simulink model "physicalModel"  (R2020b)
settings: Solver=ode3  StartTime=0.0  StopTime=10.0  FixedStep=Ts  RelTol=1e-3  EnableMultiTasking=on
undefined symbols (not defined in the file): Earth, init, Vehicle, WGS84
libraries: dynamicsLibrary x4, shared6dof x1, aerolibtransform2 x1
settings Model: Creator=dbell44  LastModifiedBy=dbell44
settings DebuggingCC: BusObjectLabelMismatch=none

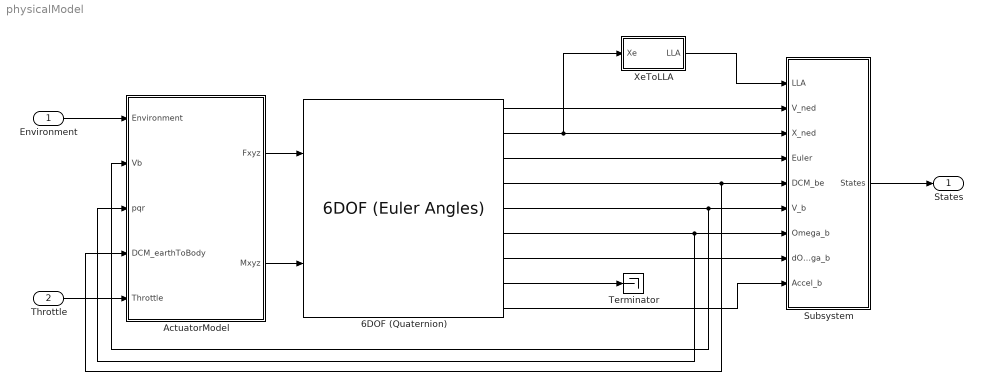
== system physicalModel ==
  Environment : Inport  OutDataTypeStr=Bus: EnvironmentBus  Interpolate=off
  Throttle : Inport  Port=2  PortDimensions=[1 4]
  6DOF (Quaternion) : shared6dof/6DOF (Euler Angles)  units=Metric (MKS)  mtype=Fixed  rep=Euler Angles  xme_0=init.posNED  Vm_0=init.vb  eul_0=init.euler  pm_0=init.angRates  mass_0=Vehicle.Airframe.mass  mass_e=0.5  mass_f=2.0  inertia=Vehicle.Airframe.inertia  inertia_e=eye(3)  inertia_f=2*eye(3)  k_quat=Vehicle.SixDOF.quatGain  vre_flag=on  abi_flag=on  aMode=aMode  xme_statename=''  Vm_statename=''  eul_statename=''  quat_statename=''  pm_statename=''  mass_statename=''
      settings: SourceProductBaseCode=AE,PW,MT,UV,VE,VP
  ActuatorModel : Subsystem
  Subsystem : Subsystem
  Terminator : Terminator
  XeToLLA : Subsystem
  States : Outport  OutDataTypeStr=Bus: StatesBus
  wires:
  ActuatorModel/1(Fxyz) -> 6DOF (Quaternion)/1
  Environment/1 -> ActuatorModel/1(Environment)
  6DOF (Quaternion)/8 -> Terminator/1
  XeToLLA/1(LLA) -> Subsystem/1(LLA)
  6DOF (Quaternion)/1 -> Subsystem/2(V_ned)
  6DOF (Quaternion)/2 -> XeToLLA/1(Xe), Subsystem/3(X_ned)
  6DOF (Quaternion)/3 -> Subsystem/4(Euler)
  6DOF (Quaternion)/5 -> ActuatorModel/2(Vb), Subsystem/6(V_b)
  6DOF (Quaternion)/6 -> Subsystem/7(Omega_b), ActuatorModel/3(pqr)
  6DOF (Quaternion)/7 -> Subsystem/8(dOmega_b)
  6DOF (Quaternion)/9 -> Subsystem/9(Accel_b)
  6DOF (Quaternion)/4 -> ActuatorModel/4(DCM_earthToBody), Subsystem/5(DCM_be)
  Subsystem/1(States) -> States/1
  Throttle/1 -> ActuatorModel/5(Throttle)
  ActuatorModel/2(Mxyz) -> 6DOF (Quaternion)/2

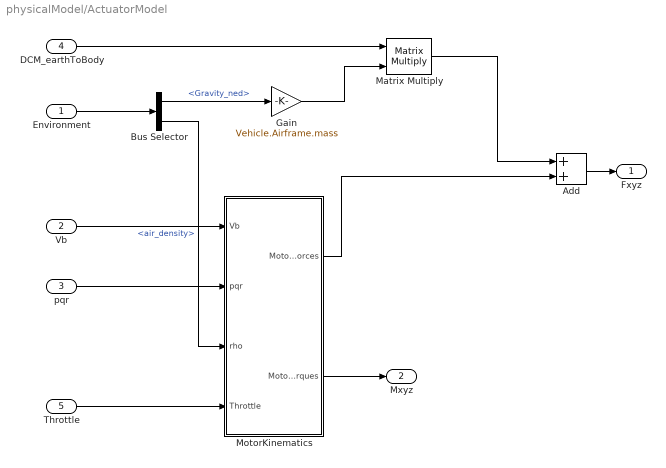
== system physicalModel/ActuatorModel ==
  Environment : Inport  OutDataTypeStr=Bus: EnvironmentBus
  Vb : Inport  Port=2
  pqr : Inport  Port=3
  DCM_earthToBody : Inport  Port=4
  Throttle : Inport  Port=5
  Add : Sum
  Bus Selector : BusSelector  OutputSignals=Gravity_ned,AtmosphereBus.air_density
  Gain : Gain  Gain=Vehicle.Airframe.mass
  Matrix Multiply : Product  Multiplication=Matrix(*)
  MotorKinematics : Subsystem
  Fxyz : Outport
  Mxyz : Outport  Port=2
  wires:
  MotorKinematics/2(MotorTorques) -> Mxyz/1
  Environment/1 -> Bus Selector/1
  Bus Selector/2 -> MotorKinematics/3(rho)  "<air_density>"
  pqr/1 -> MotorKinematics/2(pqr)
  Vb/1 -> MotorKinematics/1(Vb)
  Bus Selector/1 -> Gain/1  "<Gravity_ned>"
  DCM_earthToBody/1 -> Matrix Multiply/1
  Gain/1 -> Matrix Multiply/2
  Matrix Multiply/1 -> Add/1
  MotorKinematics/1(MotorForces) -> Add/2
  Add/1 -> Fxyz/1
  Throttle/1 -> MotorKinematics/4(Throttle)

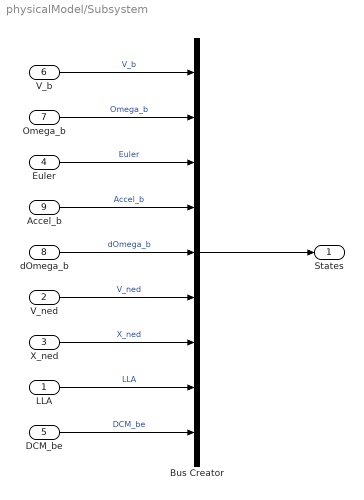
== system physicalModel/Subsystem ==
  LLA : Inport
  V_ned : Inport  Port=2
  X_ned : Inport  Port=3
  Euler : Inport  Port=4
  DCM_be : Inport  Port=5
  V_b : Inport  Port=6
  Omega_b : Inport  Port=7
  dOmega_b : Inport  Port=8
  Accel_b : Inport  Port=9
  Bus Creator : BusCreator  Inputs=9  OutDataTypeStr=Bus: StatesBus
      settings: InheritFromInputs=off
  States : Outport
  wires:
  LLA/1 -> Bus Creator/8  "LLA"
  V_ned/1 -> Bus Creator/6  "V_ned"
  X_ned/1 -> Bus Creator/7  "X_ned"
  Euler/1 -> Bus Creator/3  "Euler"
  DCM_be/1 -> Bus Creator/9  "DCM_be"
  V_b/1 -> Bus Creator/1  "V_b"
  Omega_b/1 -> Bus Creator/2  "Omega_b"
  dOmega_b/1 -> Bus Creator/5  "dOmega_b"
  Accel_b/1 -> Bus Creator/4  "Accel_b"
  Bus Creator/1 -> States/1

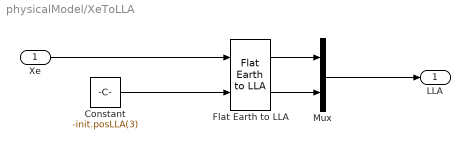
== system physicalModel/XeToLLA ==
  Xe : Inport
  Constant : Constant  Value=-init.posLLA(3)
  Flat Earth to LLA : aerolibtransform2/Flat Earth to LLA  units=Metric (MKS)  ptype=Earth (WGS84)  F=1/298.257223563  R=6378137  refPosPort=off  LL0=[0 10]  psi=0
  Mux : Mux  Inputs=2
  LLA : Outport
  wires:
  Xe/1 -> Flat Earth to LLA/1
  Mux/1 -> LLA/1
  Constant/1 -> Flat Earth to LLA/2
  Flat Earth to LLA/1 -> Mux/1
  Flat Earth to LLA/2 -> Mux/2

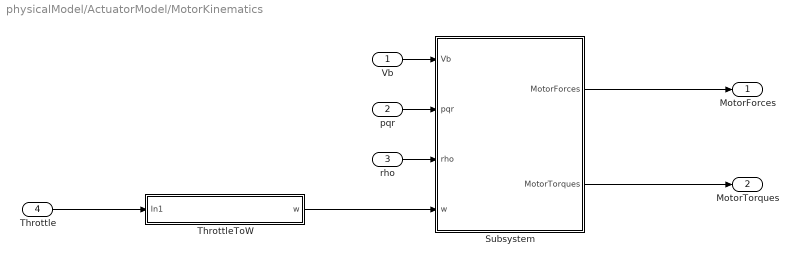
== system physicalModel/ActuatorModel/MotorKinematics ==
  Vb : Inport
  pqr : Inport  Port=2
  rho : Inport  Port=3
  Throttle : Inport  Port=4
  Subsystem : Subsystem
  ThrottleToW : Subsystem
  MotorForces : Outport
  MotorTorques : Outport  Port=2
  wires:
  pqr/1 -> Subsystem/2(pqr)
  rho/1 -> Subsystem/3(rho)
  Vb/1 -> Subsystem/1(Vb)
  Subsystem/2(MotorTorques) -> MotorTorques/1
  Subsystem/1(MotorForces) -> MotorForces/1
  Throttle/1 -> ThrottleToW/1(In1)
  ThrottleToW/1(w) -> Subsystem/4(w)

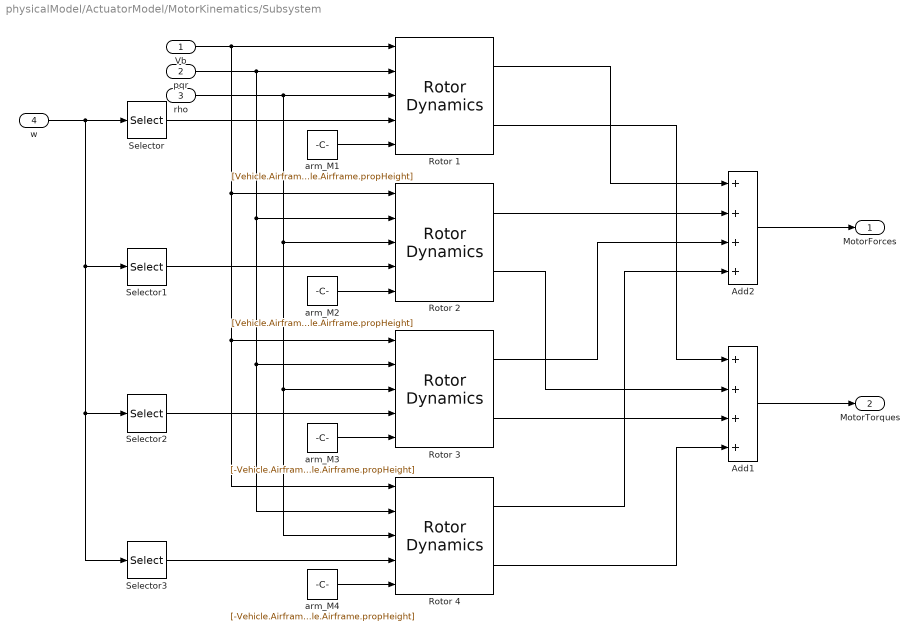
== system physicalModel/ActuatorModel/MotorKinematics/Subsystem ==
  Vb : Inport
  pqr : Inport  Port=2
  rho : Inport  Port=3
  w : Inport  Port=4
  Add1 : Sum  Inputs=++++
  Add2 : Sum  Inputs=++++
  Rotor {1..4} (4 alike) : dynamicsLibrary/Rotor Dynamics  SystemSampleTime=-1  VariantActivationTime=update diagram  Latency=0  AutoFrameSizeCalculation=off
  Selector : Selector  InputPortWidth=4  IndexOptions=Index vector (dialog)  Indices=1  OutputSizes=1
  Selector1 : Selector  InputPortWidth=4  IndexOptions=Index vector (dialog)  Indices=2  OutputSizes=1
  Selector2 : Selector  InputPortWidth=4  IndexOptions=Index vector (dialog)  Indices=3  OutputSizes=1
  Selector3 : Selector  InputPortWidth=4  IndexOptions=Index vector (dialog)  Indices=4  OutputSizes=1
  arm_M1 : Constant  Value=[Vehicle.Airframe.orthagPropDistance Vehicle.Airframe.orthagPropDistance Vehicle.Airframe.propHeight]
  arm_M2 : Constant  Value=[Vehicle.Airframe.orthagPropDistance -Vehicle.Airframe.orthagPropDistance Vehicle.Airframe.propHeight]
  arm_M3 : Constant  Value=[-Vehicle.Airframe.orthagPropDistance Vehicle.Airframe.orthagPropDistance Vehicle.Airframe.propHeight]
  arm_M4 : Constant  Value=[-Vehicle.Airframe.orthagPropDistance -Vehicle.Airframe.orthagPropDistance Vehicle.Airframe.propHeight]
  MotorForces : Outport
  MotorTorques : Outport  Port=2
  wires:
  arm_M4/1 -> Rotor 4/5
  arm_M3/1 -> Rotor 3/5
  arm_M2/1 -> Rotor 2/5
  arm_M1/1 -> Rotor 1/5
  Vb/1 -> Rotor 2/1, Rotor 4/1, Rotor 3/1, Rotor 1/1
  pqr/1 -> Rotor 4/2, Rotor 3/2, Rotor 2/2, Rotor 1/2
  Selector/1 -> Rotor 1/4
  w/1 -> Selector3/1, Selector2/1, Selector1/1, Selector/1
  Selector1/1 -> Rotor 2/4
  Selector2/1 -> Rotor 3/4
  Selector3/1 -> Rotor 4/4
  Rotor 1/1 -> Add2/1
  Rotor 2/1 -> Add2/2
  Rotor 3/1 -> Add2/3
  Rotor 4/1 -> Add2/4
  Rotor 1/2 -> Add1/1
  Rotor 2/2 -> Add1/2
  Rotor 3/2 -> Add1/3
  Rotor 4/2 -> Add1/4
  Add1/1 -> MotorTorques/1
  Add2/1 -> MotorForces/1
  rho/1 -> Rotor 4/3, Rotor 3/3, Rotor 2/3, Rotor 1/3

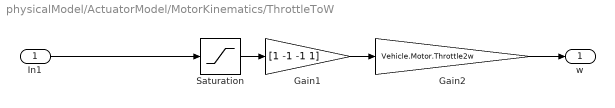
== system physicalModel/ActuatorModel/MotorKinematics/ThrottleToW ==
  In1 : Inport
  Gain1 : Gain  Gain=[1 -1 -1 1]
  Gain2 : Gain  Gain=Vehicle.Motor.Throttle2w
  Saturation : Saturate  UpperLimit=Vehicle.Motor.maxSignal  LowerLimit=Vehicle.Motor.minSignal  LinearizeAsGain=off
  w : Outport
  wires:
  In1/1 -> Saturation/1
  Saturation/1 -> Gain1/1
  Gain1/1 -> Gain2/1
  Gain2/1 -> w/1
